simulink model "EPT"  (R2019b)
settings: Solver=FixedStepDiscrete  StartTime=0.0  StopTime=5  FixedStep=0.005  RelTol=1e-3  EnableMultiTasking=on
PreLoadFcn:
  | try, model_open; catch, disp('Error occurred while executing model pre-load callback: model_open.m'); disp('Please assure that the MATLAB working directory is set to the model directory before opening.'); end
InitFcn:
  | try, model_open; catch, end
undefined symbols (not defined in the file or in its folder): Bridge, GCM, H, ln, raptor_get_param_eval, raptor_get_safe_string, raptor_xcp_function
libraries: Raptor_lib x2810, simulink x374, hdlsllib x19
(part 9 of 45)

== system EPT/Foreground_TimeBase_5ms/CHG//DCHG_PW_Control/CHG//DCHG_Current_Control/Idchg_con Soft Recovery  ==
  Idch_con : Inport
  Constant : Constant
  Delay : Delay  DelayLength=1
  Delay1 : Subsystem
  Display{1..4} (4 alike) : Display
  Latch1 : Subsystem
  Logical Operator : Logic  Operator=OR  AllPortsSameDT=off  OutDataTypeStr=boolean
  NOT : Logic  Operator=NOT  IconShape=distinctive  AllPortsSameDT=off  OutDataTypeStr=boolean
  Product1 : Product
  Relational Operator1 : RelationalOperator  OutDataTypeStr=boolean  RndMeth=Simplest
  Saturation Dynamic2 : simulink/Discontinuities/Saturation Dynamic  OutMin=[]  OutMax=[]  OutDataTypeStr=Inherit: Same as second input  OutDataType=fixdt(1, 16)  OutScaling=2^-10  DoSatur=off
  Sum : Sum  Inputs=+-
  Sum1 : Sum
  Switch : Switch  Criteria=u2 > Threshold
      settings: LockScale=on
  Switch1 : Switch  Criteria=u2 > Threshold
      settings: LockScale=on
  raptor_adjustment1 : Raptor_lib/Data Storage/raptor_adjustment  paramName='Cal_Idschg_con_Soft_recovery_TimeCount'  nameSource=Parameter  initValue=3  dataType=double  storage=Calibration  calDispType=Number  calEnum={'False', 'True'}  calGain=1.0  calOffset=0.0  calMax=inf  calMin=-inf  calFormat='-1'  calUnit=''  calHelp=''  calAccess=1  calFunction=raptor_xcp_function(gcb)  calDispHeaders=off  calColHeaders={'Col1' 'Col2' 'Col3'}  calRowHeaders={'Row1' 'Row2' 'Row3'}
      settings: SourceProductName=Raptor
  raptor_adjustment2 : Raptor_lib/Data Storage/raptor_adjustment  paramName='Cal_Idschg_con_Soft_recovery_PID_offset'  nameSource=Parameter  initValue=-0.001  dataType=double  storage=Calibration  calDispType=Number  calEnum={'False', 'True'}  calGain=1.0  calOffset=0.0  calMax=inf  calMin=-inf  calFormat='-1'  calUnit=''  calHelp=''  calAccess=1  calFunction=raptor_xcp_function(gcb)  calDispHeaders=off  calColHeaders={'Col1' 'Col2' 'Col3'}  calRowHeaders={'Row1' 'Row2' 'Row3'}
      settings: SourceProductName=Raptor
  raptor_adjustment4 : Raptor_lib/Data Storage/raptor_adjustment  paramName='Cal_Idschg_con_Soft_recovery_PID_KI'  nameSource=Parameter  initValue=0.05  dataType=double  storage=Calibration  calDispType=Number  calEnum={'False', 'True'}  calGain=1.0  calOffset=0.0  calMax=inf  calMin=-inf  calFormat='-1'  calUnit=''  calHelp=''  calAccess=1  calFunction=raptor_xcp_function(gcb)  calDispHeaders=off  calColHeaders={'Col1' 'Col2' 'Col3'}  calRowHeaders={'Row1' 'Row2' 'Row3'}
      settings: SourceProductName=Raptor
  Idchg_con : Outport
  wires:
  Saturation Dynamic2/1 -> Display4/1, Sum1/1
  Idch_con/1 -> Switch/1, Product1/2, Sum/1, Switch1/1, Relational Operator1/1
  Sum/1 -> Display3/1
  Switch/1 -> Sum/2
  Product1/1 -> Saturation Dynamic2/2
  raptor_adjustment2/1 -> Saturation Dynamic2/3, Saturation Dynamic2/1
  Sum1/1 -> Delay/1
  raptor_adjustment4/1 -> Product1/1
  Switch1/1 -> Sum1/2, Display2/1, Display1/1, Idchg_con/1
  Delay/1 -> Switch1/3, Switch/3, Relational Operator1/2
  Relational Operator1/1 -> Logical Operator/1
  Constant/1 -> Delay1/1(Condition)
  Latch1/1(Output) -> NOT/1
  Logical Operator/1 -> Switch1/2, Switch/2
  raptor_adjustment1/1 -> Delay1/2(TimeCount)
  Delay1/1(Output) -> Latch1/1(Latch)
  NOT/1 -> Logical Operator/2

== system EPT/Foreground_TimeBase_5ms/CHG//DCHG_PW_Control/CHG//DCHG_Current_Control/Soft Recovery ==
  HV_Current : Inport
  Idchg_con : Inport  Port=2
  Add4 : Sum  Inputs=+-
  Delay : Delay  DelayLength=1
  Delay1 : Delay  DelayLength=1
  Gain1 : Gain  Gain=1.5
  IsNegative : simulink/Logic and Bit Operations/Compare To Zero  relop=<  OutDataTypeStr=boolean
  IsPositive : simulink/Logic and Bit Operations/Compare To Zero  relop=>  OutDataTypeStr=boolean
  Logical Operator3 : Logic  AllPortsSameDT=off  OutDataTypeStr=boolean
  Logical Operator4 : Logic  AllPortsSameDT=off  OutDataTypeStr=boolean
  Logical Operator5 : Logic  Operator=NOR  AllPortsSameDT=off  OutDataTypeStr=boolean
  Relational Operator2 : RelationalOperator  Operator=<=  OutDataTypeStr=boolean  RndMeth=Simplest
  Relational Operator3 : RelationalOperator  OutDataTypeStr=boolean  RndMeth=Simplest
  Saturation Dynamic2 : simulink/Discontinuities/Saturation Dynamic  OutMin=[]  OutMax=[]  OutDataTypeStr=Inherit: Same as second input  OutDataType=fixdt(1, 16)  OutScaling=2^-10  DoSatur=off
  Subsystem2 : Subsystem
  raptor_adjustment : Raptor_lib/Data Storage/raptor_adjustment  paramName='Cal_Recovery_Time_Ft'  nameSource=Parameter  initValue=0.066  dataType=double  storage=Calibration  calDispType=Number  calEnum={'False', 'True'}  calGain=1.0  calOffset=0.0  calMax=inf  calMin=-inf  calFormat='-1'  calUnit=''  calHelp=''  calAccess=1  calFunction=raptor_xcp_function(gcb)  calDispHeaders=off  calColHeaders={'Col1' 'Col2' 'Col3'}  calRowHeaders={'Row1' 'Row2' 'Row3'}
      settings: SourceProductName=Raptor
  Idchg_exp : Outport
  wires:
  Gain1/1 -> Saturation Dynamic2/3, Relational Operator2/2
  Idchg_con/1 -> Relational Operator3/2, Saturation Dynamic2/1, Gain1/1, Subsystem2/1(Idchg_con), Add4/2
  IsNegative/1 -> Logical Operator4/1
  Logical Operator4/1 -> Logical Operator5/2
  IsPositive/1 -> Logical Operator3/1
  Logical Operator5/1 -> Subsystem2/Enable
  Logical Operator3/1 -> Logical Operator5/1
  Relational Operator3/1 -> Delay1/1
  Saturation Dynamic2/1 -> Relational Operator2/1, Relational Operator3/1, Idchg_exp/1
  Subsystem2/1(Gain_Integral) -> Saturation Dynamic2/2
  Relational Operator2/1 -> Delay/1
  HV_Current/1 -> Add4/1
  raptor_adjustment/1 -> Subsystem2/3(Recovery_Time_Ft)
  Delay/1 -> Logical Operator3/2
  Delay1/1 -> Logical Operator4/2
  Add4/1 -> Subsystem2/2(Delta_Idchg), IsNegative/1, IsPositive/1

== system EPT/Foreground_TimeBase_5ms/CHG//DCHG_PW_Control/Coulomb Counting Algorithm/Coulomb Counting Algorithm ==
  Ampere input : Inport
  RC input : Inport  Port=2
  20ms : Subsystem
  Constant6 : Constant  Value=4
  CountTrigger : Subsystem
  wires:
  CountTrigger/1(Tirgger) -> 20ms/Trigger
  Constant6/1 -> CountTrigger/1(Counter)
  RC input/1 -> 20ms/2(RC input)
  Ampere input/1 -> 20ms/1(Ampere input)

== system EPT/Foreground_TimeBase_5ms/CHG//DCHG_PW_Control/Coulomb Counting Algorithm/Delay ==
  Condition : Inport
  TimeCount : Inport  Port=2
  Constant10 : Constant
  Constant11 : Constant  Value=0
  Constant8 : Constant  Value=0
  CycleTrigger : Subsystem
  Switch2 : Switch  Threshold=1
  Switch3 : Switch  Threshold=1
  Unit Delay1 : UnitDelay  SampleTime=-1  HasFrameUpgradeWarning=on
  Unit Delay2 : UnitDelay  SampleTime=-1  HasFrameUpgradeWarning=on
  Output : Outport  VectorParamsAs1DForOutWhenUnconnected=off
  wires:
  TimeCount/1 -> CycleTrigger/2(In2)
  Condition/1 -> Switch3/2
  CycleTrigger/1(Trigger) -> Switch2/2, Unit Delay1/1
  Constant8/1 -> Switch2/1
  Constant10/1 -> Switch2/3
  Switch3/1 -> CycleTrigger/1(In1)
  Constant11/1 -> Switch3/3
  Unit Delay2/1 -> Switch3/1
  Switch2/1 -> Unit Delay2/1
  Unit Delay1/1 -> Output/1

== system EPT/Foreground_TimeBase_5ms/CHG//DCHG_PW_Control/Coulomb Counting Algorithm/Latch ==
  Latch : Inport
  Reset : Inport  Port=2
  Switch1 : Switch  Criteria=u2 > Threshold
  Switch3 : Switch  Criteria=u2 > Threshold
  Unit Delay1 : UnitDelay  SampleTime=-1  HasFrameUpgradeWarning=on
  Output : Outport  VectorParamsAs1DForOutWhenUnconnected=off
  wires:
  Unit Delay1/1 -> Switch1/3
  Switch3/1 -> Output/1, Unit Delay1/1
  Reset/1 -> Switch3/2
  Latch/1 -> Switch1/1, Switch1/2
  Switch1/1 -> Switch3/3

== system EPT/Foreground_TimeBase_5ms/CHG//DCHG_PW_Control/Coulomb Counting Algorithm/WH  ==
  Ampere input : Inport
  Voltage input : Inport  Port=2
  WH input : Inport  Port=3
  Enable : EnablePort
  20ms : Subsystem
  Constant6 : Constant  Value=4
  CountTrigger : Subsystem
  WH Output : Outport  VectorParamsAs1DForOutWhenUnconnected=off
  wires:
  Voltage input/1 -> 20ms/2(Voltage input)
  Ampere input/1 -> 20ms/1(Ampere input)
  20ms/1(WH Output) -> WH Output/1
  Constant6/1 -> CountTrigger/1(Counter)
  CountTrigger/1(Tirgger) -> 20ms/Trigger
  WH input/1 -> 20ms/3(WH Input)

== system EPT/Foreground_TimeBase_5ms/CHG//DCHG_PW_Control/EOC/Delay1 ==
  Condition : Inport
  TimeCount : Inport  Port=2
  Constant10 : Constant
  Constant11 : Constant  Value=0
  Constant8 : Constant  Value=0
  CycleTrigger : Subsystem
  Switch2 : Switch  Threshold=1
  Switch3 : Switch  Threshold=1
  Unit Delay1 : UnitDelay  SampleTime=-1  HasFrameUpgradeWarning=on
  Unit Delay2 : UnitDelay  SampleTime=-1  HasFrameUpgradeWarning=on
  Output : Outport  VectorParamsAs1DForOutWhenUnconnected=off
  wires:
  Unit Delay1/1 -> Output/1
  Switch2/1 -> Unit Delay2/1
  Unit Delay2/1 -> Switch3/1
  Constant11/1 -> Switch3/3
  Switch3/1 -> CycleTrigger/1(In1)
  Constant10/1 -> Switch2/3
  Constant8/1 -> Switch2/1
  CycleTrigger/1(Trigger) -> Unit Delay1/1, Switch2/2
  Condition/1 -> Switch3/2
  TimeCount/1 -> CycleTrigger/2(In2)

== system EPT/Foreground_TimeBase_5ms/CHG//DCHG_PW_Control/EOC/EOC_Table ==
  Abs : Abs
  Add : Sum
  raptor_adjustment1 : Raptor_lib/Data Storage/raptor_adjustment  paramName='EOC_Offset'  nameSource=Parameter  initValue=0.0  dataType=double  storage=Calibration  calDispType=Number  calEnum={'False', 'True'}  calGain=1.0  calOffset=0.0  calMax=inf  calMin=-inf  calFormat='-1'  calUnit=''  calHelp=''  calAccess=1  calFunction=raptor_xcp_function(gcb)  calDispHeaders=off  calColHeaders={'Col1' 'Col2' 'Col3'}  calRowHeaders={'Row1' 'Row2' 'Row3'}
      settings: SourceProductName=Raptor
  raptor_data_read9 : Raptor_lib/Data Storage/raptor_data_read  dataName='EPT_BPOBU_CURR'  dataShape=Scalar  idxSource=Input  idxRow=1  idxCol=1
      settings: SourceProductName=Raptor
  raptor_table_1d1 : Raptor_lib/Table Lookup/raptor_table_1d  dataName='Amp2EOCVoltage_V2'  initValue=|  dataType=double  storage=Calibration  initValueX=|  dataTypeXY=double  storageXY=Calibration  calVisible=on  showTable=on  calGain=1  calOffset=0.0  calMax=Inf  calMin=-Inf  calFormat='-1'  calUnit=''  calHelp=''  showBreakpoint=on  dataNameX=[]  calGainX=1.0  calOffsetX=0.0  calMaxX=Inf  calMinX=-Inf  calFormatX='-1'  calUnitX=''  calHelpX=''  calAccess=1  calFunction=raptor_xcp_function(gcb)  measureEnable=off  mName=[raptor_get_param_eval(gcb,'dataName'), '_Output']
      initValue=|
      | [3.4
      | 3.45
      | 3.48
      | 3.5
      | 3.52
      | 3.54
      | 3.56
      | 3.58
      | 3.6
      | ]
      initValueX=|
      | [0
      | 5
      | 10
      | 15
      | 20
      | 25
      | 30
      | 40
      | 50
      | ]
      settings: SourceProductName=Raptor
  raptor_table_1d2 : Raptor_lib/Table Lookup/raptor_table_1d  dataName='Amp2EOCVoltage'  initValue=|  dataType=double  storage=Calibration  initValueX=|  dataTypeXY=double  storageXY=Calibration  calVisible=on  showTable=on  calGain=1  calOffset=0.0  calMax=Inf  calMin=-Inf  calFormat='-1'  calUnit=''  calHelp=''  showBreakpoint=on  dataNameX=[]  calGainX=1.0  calOffsetX=0.0  calMaxX=Inf  calMinX=-Inf  calFormatX='-1'  calUnitX=''  calHelpX=''  calAccess=1  calFunction=raptor_xcp_function(gcb)  measureEnable=off  mName=[raptor_get_param_eval(gcb,'dataName'), '_Output']
      initValue=|
      | [3.34
      | 3.35
      | 3.36
      | 3.39
      | 3.4
      | 3.41
      | 3.42
      | 3.45
      | 3.5
      | 3.5
      | 3.5
      | 3.5
      | 
      | ]
      initValueX=|
      | [0
      | 2.5
      | 5
      | 7.5
      | 10
      | 12.5
      | 15
      | 20
      | 25
      | 37.5
      | 50
      | 100
      | ]*3
      settings: SourceProductName=Raptor
  CellVoltage : Outport  VectorParamsAs1DForOutWhenUnconnected=off
  wires:
  raptor_table_1d1/1 -> Add/1
  raptor_adjustment1/1 -> Add/2
  raptor_data_read9/1 -> Abs/1
  Add/1 -> CellVoltage/1
  Abs/1 -> raptor_table_1d1/1

== system EPT/Foreground_TimeBase_5ms/CHG//DCHG_PW_Control/EOC/Latch1 ==
  Latch : Inport
  Reset : Inport  Port=2
  Switch1 : Switch  Criteria=u2 > Threshold
  Switch3 : Switch  Criteria=u2 > Threshold
  Unit Delay1 : UnitDelay  SampleTime=-1  HasFrameUpgradeWarning=on
  Output : Outport  VectorParamsAs1DForOutWhenUnconnected=off
  wires:
  Unit Delay1/1 -> Switch1/3
  Switch3/1 -> Output/1, Unit Delay1/1
  Reset/1 -> Switch3/2
  Latch/1 -> Switch1/1, Switch1/2
  Switch1/1 -> Switch3/3

== system EPT/Foreground_TimeBase_5ms/CHG//DCHG_PW_Control/EOD/Delay1 ==
  Condition : Inport
  TimeCount : Inport  Port=2
  Constant10 : Constant
  Constant11 : Constant  Value=0
  Constant8 : Constant  Value=0
  CycleTrigger : Subsystem
  Switch2 : Switch  Threshold=1
  Switch3 : Switch  Threshold=1
  Unit Delay1 : UnitDelay  SampleTime=-1  HasFrameUpgradeWarning=on
  Unit Delay2 : UnitDelay  SampleTime=-1  HasFrameUpgradeWarning=on
  Output : Outport  VectorParamsAs1DForOutWhenUnconnected=off
  wires:
  Unit Delay1/1 -> Output/1
  Switch2/1 -> Unit Delay2/1
  Unit Delay2/1 -> Switch3/1
  Constant11/1 -> Switch3/3
  Switch3/1 -> CycleTrigger/1(In1)
  Constant10/1 -> Switch2/3
  Constant8/1 -> Switch2/1
  CycleTrigger/1(Trigger) -> Unit Delay1/1, Switch2/2
  Condition/1 -> Switch3/2
  TimeCount/1 -> CycleTrigger/2(In2)

== system EPT/Foreground_TimeBase_5ms/CHG//DCHG_PW_Control/EOD/EOD_Table ==
  Abs : Abs
  Display : Display
  Subtract : Sum  Inputs=+-
  raptor_adjustment : Raptor_lib/Data Storage/raptor_adjustment  paramName='EOD_Offset'  nameSource=Parameter  initValue=0.1  dataType=double  storage=Calibration  calDispType=Number  calEnum={'False', 'True'}  calGain=1.0  calOffset=0.0  calMax=inf  calMin=-inf  calFormat='-1'  calUnit=''  calHelp=''  calAccess=1  calFunction=raptor_xcp_function(gcb)  calDispHeaders=off  calColHeaders={'Col1' 'Col2' 'Col3'}  calRowHeaders={'Row1' 'Row2' 'Row3'}
      settings: SourceProductName=Raptor
  raptor_data_read9 : Raptor_lib/Data Storage/raptor_data_read  dataName='EPT_BPOBU_CURR'  dataShape=Scalar  idxSource=Input  idxRow=1  idxCol=1
      settings: SourceProductName=Raptor
  raptor_table_1d1 : Raptor_lib/Table Lookup/raptor_table_1d  dataName='Amp2EODVoltage'  initValue=|  dataType=double  storage=Calibration  initValueX=|  dataTypeXY=double  storageXY=Calibration  calVisible=on  showTable=on  calGain=1  calOffset=0.0  calMax=Inf  calMin=-Inf  calFormat='-1'  calUnit=''  calHelp=''  showBreakpoint=on  dataNameX=[]  calGainX=1.0  calOffsetX=0.0  calMaxX=Inf  calMinX=-Inf  calFormatX='-1'  calUnitX=''  calHelpX=''  calAccess=1  calFunction=raptor_xcp_function(gcb)  measureEnable=off  mName=[raptor_get_param_eval(gcb,'dataName'), '_Output']
      initValue=|
      | [3.05
      | 2.99
      | 2.94
      | 2.89
      | 2.86
      | 2.82
      | 2.79
      | 2.72
      | 2.65
      | 2.6
      | 2.6
      | 2.6
      | 2.6
      | ]
      initValueX=|
      | [0
      | 5
      | 10
      | 15
      | 20
      | 25
      | 30
      | 40
      | 50
      | 100
      | 150
      | 200
      | 300
      | ]
      settings: SourceProductName=Raptor
  CellVoltage : Outport  VectorParamsAs1DForOutWhenUnconnected=off
  wires:
  Subtract/1 -> CellVoltage/1, Display/1
  raptor_table_1d1/1 -> Subtract/1
  raptor_adjustment/1 -> Subtract/2
  raptor_data_read9/1 -> Abs/1
  Abs/1 -> raptor_table_1d1/1

== system EPT/Foreground_TimeBase_5ms/CHG//DCHG_PW_Control/EOD/Latch1 ==
  Latch : Inport
  Reset : Inport  Port=2
  Switch1 : Switch  Criteria=u2 > Threshold
  Switch3 : Switch  Criteria=u2 > Threshold
  Unit Delay1 : UnitDelay  SampleTime=-1  HasFrameUpgradeWarning=on
  Output : Outport  VectorParamsAs1DForOutWhenUnconnected=off
  wires:
  Unit Delay1/1 -> Switch1/3
  Switch3/1 -> Output/1, Unit Delay1/1
  Reset/1 -> Switch3/2
  Latch/1 -> Switch1/1, Switch1/2
  Switch1/1 -> Switch3/3

== system EPT/Foreground_TimeBase_5ms/CHG//DCHG_PW_Control/Enhanced Coulomb Counting Algorithm/Coulomb Counting ==
  Ib : Inport
  Ah Input : Inport  Port=2
  20ms : Subsystem
  Constant6 : Constant  Value=4
  CountTrigger : Subsystem
  Gain2 : Gain  Gain=-1
  Ah Output : Outport
  wires:
  Ah Input/1 -> 20ms/2(Delta_DoD)
  Constant6/1 -> CountTrigger/1(Counter)
  CountTrigger/1(Tirgger) -> 20ms/Trigger
  20ms/1(Delta DoD) -> Ah Output/1
  Ib/1 -> Gain2/1
  Gain2/1 -> 20ms/1(Ib)

== system EPT/Foreground_TimeBase_5ms/CHG//DCHG_PW_Control/Enhanced Coulomb Counting Algorithm/Init Enhanced Coulomb Counting Algorithm ==
  Enable : EnablePort
  raptor_adjustment : Raptor_lib/Data Storage/raptor_adjustment  paramName='Cal_DOD_t0'  nameSource=Parameter  initValue=0.00  dataType=double  storage=Calibration  calDispType=Number  calEnum={'False', 'True'}  calGain=1.0  calOffset=0.0  calMax=inf  calMin=-inf  calFormat='-1'  calUnit=''  calHelp=''  calAccess=1  calFunction=raptor_xcp_function(gcb)  calDispHeaders=off  calColHeaders={'Col1' 'Col2' 'Col3'}  calRowHeaders={'Row1' 'Row2' 'Row3'}
      settings: SourceProductName=Raptor
  raptor_adjustment1 : Raptor_lib/Data Storage/raptor_adjustment  paramName='Cal_SOH'  nameSource=Parameter  initValue=0.00  dataType=double  storage=Calibration  calDispType=Number  calEnum={'False', 'True'}  calGain=1.0  calOffset=0.0  calMax=inf  calMin=-inf  calFormat='-1'  calUnit=''  calHelp=''  calAccess=1  calFunction=raptor_xcp_function(gcb)  calDispHeaders=off  calColHeaders={'Col1' 'Col2' 'Col3'}  calRowHeaders={'Row1' 'Row2' 'Row3'}
      settings: SourceProductName=Raptor
  raptor_data_write1 : Raptor_lib/Data Storage/raptor_data_write  dataName='SOH'  dataShape=Scalar  idxSource=Input Port  idxRow=1  idxCol=1
      settings: SourceProductName=Raptor
  raptor_data_write2 : Raptor_lib/Data Storage/raptor_data_write  dataName='DOD_t0'  dataShape=Scalar  idxSource=Input Port  idxRow=1  idxCol=1
      settings: SourceProductName=Raptor
  wires:
  raptor_adjustment/1 -> raptor_data_write2/1
  raptor_adjustment1/1 -> raptor_data_write1/1

== system EPT/Foreground_TimeBase_5ms/CHG//DCHG_PW_Control/Enhanced Coulomb Counting Algorithm Backup/Coulomb Counting1 ==
  Ib : Inport
  Ah Input : Inport  Port=2
  20ms : Subsystem
  Constant6 : Constant  Value=4
  CountTrigger : Subsystem
  Gain2 : Gain  Gain=-1
  Ah Output : Outport
  wires:
  Gain2/1 -> 20ms/1(Ib)
  Ib/1 -> Gain2/1
  20ms/1(Delta DoD) -> Ah Output/1
  CountTrigger/1(Tirgger) -> 20ms/Trigger
  Constant6/1 -> CountTrigger/1(Counter)
  Ah Input/1 -> 20ms/2(Delta_DoD)

== system EPT/Foreground_TimeBase_5ms/CHG//DCHG_PW_Control/SWU Power Divider/PWCU ==
  Constant1 : Constant
  Constant10 : Constant  Value=70
  Constant3 : Constant  Value=50
  Constant9 : Constant
  Latch1 : Subsystem
  Latch2 : Subsystem
  Product{2..6} (5 alike) : Product
  Relational Operator1 : RelationalOperator  Operator=>  OutDataTypeStr=boolean  RndMeth=Simplest
  Relational Operator2 : RelationalOperator  Operator=>  OutDataTypeStr=boolean  RndMeth=Simplest
  Relational Operator3 : RelationalOperator  Operator=<=  OutDataTypeStr=boolean  RndMeth=Simplest
  Relational Operator4 : RelationalOperator  Operator=<=  OutDataTypeStr=boolean  RndMeth=Simplest
  Saturation Dynamic : simulink/Discontinuities/Saturation Dynamic  OutMin=[]  OutMax=[]  OutDataTypeStr=Inherit: Same as second input  OutDataType=fixdt(1, 16)  OutScaling=2^-10  DoSatur=off
  Subtract3 : Sum
  Subtract4 : Sum  Inputs=+-
  Subtract5 : Sum
  Subtract6 : Sum  Inputs=+-
  Switch1 : Switch  Criteria=u2 > Threshold
  Total PW. : Constant  Value=9
  raptor_adjustment : Raptor_lib/Data Storage/raptor_adjustment  paramName='Cal_OBU_RSOC_Lower_Limit_error'  nameSource=Parameter  initValue=0.02  dataType=double  storage=Calibration  calDispType=Number  calEnum={'False', 'True'}  calGain=1.0  calOffset=0.0  calMax=inf  calMin=-inf  calFormat='-1'  calUnit=''  calHelp=''  calAccess=1  calFunction=raptor_xcp_function(gcb)  calDispHeaders=off  calColHeaders={'Col1' 'Col2' 'Col3'}  calRowHeaders={'Row1' 'Row2' 'Row3'}
      settings: SourceProductName=Raptor
  raptor_adjustment2 : Raptor_lib/Data Storage/raptor_adjustment  paramName='Cal_OBU_RSOC_Upper_Limit_error'  nameSource=Parameter  initValue=0.02  dataType=double  storage=Calibration  calDispType=Number  calEnum={'False', 'True'}  calGain=1.0  calOffset=0.0  calMax=inf  calMin=-inf  calFormat='-1'  calUnit=''  calHelp=''  calAccess=1  calFunction=raptor_xcp_function(gcb)  calDispHeaders=off  calColHeaders={'Col1' 'Col2' 'Col3'}  calRowHeaders={'Row1' 'Row2' 'Row3'}
      settings: SourceProductName=Raptor
  raptor_data_read1 : Raptor_lib/Data Storage/raptor_data_read  dataName='SWCU_BPSWU_POUT_MAX'  dataShape=Scalar  idxSource=Input  idxRow=1  idxCol=1
      settings: SourceProductName=Raptor
  raptor_data_read3 : Raptor_lib/Data Storage/raptor_data_read  dataName='EPT_BPOBU_SOC'  dataShape=Scalar  idxSource=Input  idxRow=1  idxCol=1
      settings: SourceProductName=Raptor
  raptor_data_write7 : Raptor_lib/Data Storage/raptor_data_write  dataName='EPT_SWCU_POUT_CMD'  dataShape=Scalar  idxSource=Input Port  idxRow=1  idxCol=1
      settings: SourceProductName=Raptor
  raptor_override3 : Raptor_lib/Data Storage/raptor_override  paramName='Cal_OBU_ROSC'  nameSource=Parameter  measurement=None  calDispType=Number  calEnum={'False', 'True'}  calGain=1.0  calOffset=0.0  calMax=inf  calMin=-inf  calFormat='-1'  calUnit=''  calHelp=''  calAccess=1  calFunction=[raptor_xcp_function(gcb) '|' raptor_get_param_eval(gcb, 'paramName') '_Override']
      settings: SourceProductName=Raptor
  raptor_table_1d : Raptor_lib/Table Lookup/raptor_table_1d  dataName='OBU_SOC2SWCU_PW'  initValue="[9 9 7.5  7.5 3.6 3.6 3.6]"  dataType=double  storage=Calibration  initValueX=[0 50 50 55 65 70 75]  dataTypeXY=double  storageXY=Calibration  calVisible=on  showTable=on  calGain=1.0  calOffset=0.0  calMax=Inf  calMin=-Inf  calFormat='-1'  calUnit=''  calHelp=''  showBreakpoint=on  dataNameX=[]  calGainX=1.0  calOffsetX=0.0  calMaxX=Inf  calMinX=-Inf  calFormatX='-1'  calUnitX=''  calHelpX=''  calAccess=1  calFunction=raptor_xcp_function(gcb)  measureEnable=off  mName=[raptor_get_param_eval(gcb,'dataName'), '_Output']
      settings: SourceProductName=Raptor
  wires:
  Product5/1 -> Relational Operator4/2
  Relational Operator3/1 -> Latch1/1(Latch)
  Product4/1 -> Relational Operator1/2
  Subtract3/1 -> Product4/2
  Relational Operator4/1 -> Latch2/1(Latch)
  Product3/1 -> Relational Operator3/2
  raptor_adjustment/1 -> Subtract3/2, Subtract4/2
  raptor_adjustment2/1 -> Subtract5/2, Subtract6/2
  Relational Operator1/1 -> Latch1/2(Reset)
  Latch2/1(Output) -> Product2/2
  Product2/1 -> Switch1/3
  Constant9/1 -> Subtract5/1, Subtract6/1
  raptor_override3/1 -> Relational Operator2/1, Relational Operator4/1, Relational Operator3/1, Relational Operator1/1, raptor_table_1d/1
  Relational Operator2/1 -> Latch2/2(Reset)
  raptor_data_read3/1 -> raptor_override3/1
  Constant3/1 -> Product4/1, Product3/1
  Subtract6/1 -> Product5/2
  raptor_table_1d/1 -> Product2/1
  Constant10/1 -> Product6/1, Product5/1
  Product6/1 -> Relational Operator2/2
  Subtract5/1 -> Product6/2
  Subtract4/1 -> Product3/2
  Latch1/1(Output) -> Switch1/2
  Total PW./1 -> Switch1/1
  Constant1/1 -> Subtract3/1, Subtract4/1
  Switch1/1 -> Saturation Dynamic/2
  Saturation Dynamic/1 -> raptor_data_write7/1
  raptor_data_read1/1 -> Saturation Dynamic/1

== system EPT/Foreground_TimeBase_5ms/E//W /BP-OBU_E//W/BP-OBU_E//W ==
  "CMU_Work " : Inport
  BP-OBU_Fault_G4 : Subsystem
  BP-OBU_Warning/Fault_G1 : Subsystem
  BP-OBU_Warning/Fault_G2 : Subsystem
  BP-OBU_Warning/Fault_G3 : Subsystem
  BP-OBU_Warning/Fault_G5 : Subsystem
  wires:
  "CMU_Work "/1 -> BP-OBU_Fault_G4/1("CMU_Work "), BP-OBU_Warning/Fault_G2/Enable, BP-OBU_Warning/Fault_G1/Enable

== system EPT/Foreground_TimeBase_5ms/E//W /BP-OBU_E//W/Delay ==
  Condition : Inport
  TimeCount : Inport  Port=2
  Constant10 : Constant
  Constant11 : Constant  Value=0
  Constant8 : Constant  Value=0
  CycleTrigger : Subsystem
  Switch2 : Switch  Threshold=1
  Switch3 : Switch  Threshold=1
  Unit Delay1 : UnitDelay  SampleTime=-1  HasFrameUpgradeWarning=on
  Unit Delay2 : UnitDelay  SampleTime=-1  HasFrameUpgradeWarning=on
  Output : Outport  VectorParamsAs1DForOutWhenUnconnected=off
  wires:
  TimeCount/1 -> CycleTrigger/2(In2)
  Condition/1 -> Switch3/2
  CycleTrigger/1(Trigger) -> Switch2/2, Unit Delay1/1
  Constant8/1 -> Switch2/1
  Constant10/1 -> Switch2/3
  Switch3/1 -> CycleTrigger/1(In1)
  Constant11/1 -> Switch3/3
  Unit Delay2/1 -> Switch3/1
  Switch2/1 -> Unit Delay2/1
  Unit Delay1/1 -> Output/1

== system EPT/Foreground_TimeBase_5ms/E//W /BP-OBU_E//W/Latch ==
  Latch : Inport
  Reset : Inport  Port=2
  Switch1 : Switch  Criteria=u2 > Threshold
  Switch3 : Switch  Criteria=u2 > Threshold
  Unit Delay1 : UnitDelay  SampleTime=-1  HasFrameUpgradeWarning=on
  Output : Outport  VectorParamsAs1DForOutWhenUnconnected=off
  wires:
  Unit Delay1/1 -> Switch1/3
  Switch3/1 -> Output/1, Unit Delay1/1
  Reset/1 -> Switch3/2
  Latch/1 -> Switch1/1, Switch1/2
  Switch1/1 -> Switch3/3

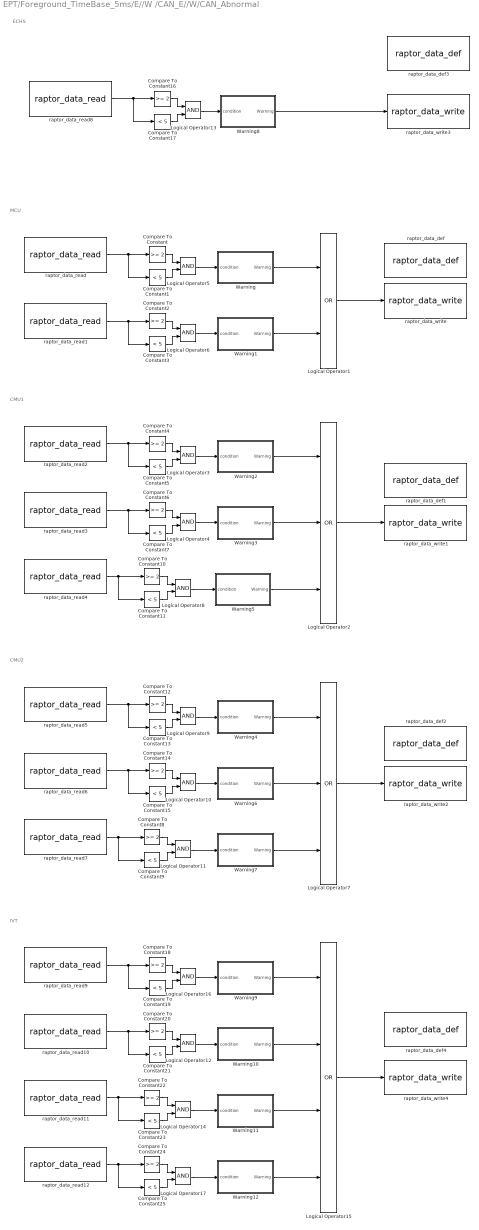
== system EPT/Foreground_TimeBase_5ms/E//W /CAN_E//W/CAN_Abnormal ==
  note: MCU
  note: CMU1
  note: CMU2
  note: ECHS
  note: IVT
  Compare To Constant{,2,4,6,8,10,12,14,16,18,20,22,24} (13 alike) : simulink/Logic and Bit Operations/Compare To Constant  relop=>=  const=2  OutDataTypeStr=boolean
  Compare To Constant{1,3,5,7,9,11,13,15,17,19,21,23,25} (13 alike) : simulink/Logic and Bit Operations/Compare To Constant  relop=<  const=5  OutDataTypeStr=boolean
  Logical Operator1 : Logic  Operator=OR  AllPortsSameDT=off  OutDataTypeStr=boolean
  Logical Operator{3..6,8..14,16..17} (13 alike) : Logic  AllPortsSameDT=off  OutDataTypeStr=boolean
  Logical Operator15 : Logic  Operator=OR  Inputs=4  AllPortsSameDT=off  OutDataTypeStr=boolean
  Logical Operator2 : Logic  Operator=OR  Inputs=3  AllPortsSameDT=off  OutDataTypeStr=boolean
  Logical Operator7 : Logic  Operator=OR  Inputs=3  AllPortsSameDT=off  OutDataTypeStr=boolean
  Warning : Subsystem
  Warning1 : Subsystem
  Warning10 : Subsystem
  Warning11 : Subsystem
  Warning12 : Subsystem
  Warning2 : Subsystem
  Warning3 : Subsystem
  Warning4 : Subsystem
  Warning5 : Subsystem
  Warning6 : Subsystem
  Warning7 : Subsystem
  Warning8 : Subsystem
  Warning9 : Subsystem
  raptor_data_def : Raptor_lib/Data Storage/raptor_data_def  dataName='CAN_Abnormal_MCU'  initValue=0  dataType=boolean  storage=Volatile (RAM)  calVisible=on  calType=Measurement  calDispType=Number  calEnum={'False', 'True'}  calGain=1.0  calOffset=0  calMin=-inf  calMax=inf  calFormat='-1'  calUnit=''  calHelp=''  calAccess=1  calFunction=raptor_xcp_function(gcb)  calDispHeaders=off  calColHeaders={'Col1' 'Col2' 'Col3'}  calRowHeaders={'Row1' 'Row2' 'Row3'}
      settings: SourceProductName=Raptor
  raptor_data_def1 : Raptor_lib/Data Storage/raptor_data_def  dataName='CAN_Abnormal_CMU1'  initValue=0  dataType=boolean  storage=Volatile (RAM)  calVisible=on  calType=Measurement  calDispType=Number  calEnum={'False', 'True'}  calGain=1.0  calOffset=0  calMin=-inf  calMax=inf  calFormat='-1'  calUnit=''  calHelp=''  calAccess=1  calFunction=raptor_xcp_function(gcb)  calDispHeaders=off  calColHeaders={'Col1' 'Col2' 'Col3'}  calRowHeaders={'Row1' 'Row2' 'Row3'}
      settings: SourceProductName=Raptor
  raptor_data_def2 : Raptor_lib/Data Storage/raptor_data_def  dataName='CAN_Abnormal_CMU2'  initValue=0  dataType=boolean  storage=Volatile (RAM)  calVisible=on  calType=Measurement  calDispType=Number  calEnum={'False', 'True'}  calGain=1.0  calOffset=0  calMin=-inf  calMax=inf  calFormat='-1'  calUnit=''  calHelp=''  calAccess=1  calFunction=raptor_xcp_function(gcb)  calDispHeaders=off  calColHeaders={'Col1' 'Col2' 'Col3'}  calRowHeaders={'Row1' 'Row2' 'Row3'}
      settings: SourceProductName=Raptor
  raptor_data_def3 : Raptor_lib/Data Storage/raptor_data_def  dataName='CAN_Abnormal_ECHS'  initValue=0  dataType=boolean  storage=Volatile (RAM)  calVisible=on  calType=Measurement  calDispType=Number  calEnum={'False', 'True'}  calGain=1.0  calOffset=0  calMin=-inf  calMax=inf  calFormat='-1'  calUnit=''  calHelp=''  calAccess=1  calFunction=raptor_xcp_function(gcb)  calDispHeaders=off  calColHeaders={'Col1' 'Col2' 'Col3'}  calRowHeaders={'Row1' 'Row2' 'Row3'}
      settings: SourceProductName=Raptor
  raptor_data_def4 : Raptor_lib/Data Storage/raptor_data_def  dataName='CAN_Abnormal_IVT'  initValue=0  dataType=boolean  storage=Volatile (RAM)  calVisible=on  calType=Measurement  calDispType=Number  calEnum={'False', 'True'}  calGain=1.0  calOffset=0  calMin=-inf  calMax=inf  calFormat='-1'  calUnit=''  calHelp=''  calAccess=1  calFunction=raptor_xcp_function(gcb)  calDispHeaders=off  calColHeaders={'Col1' 'Col2' 'Col3'}  calRowHeaders={'Row1' 'Row2' 'Row3'}
      settings: SourceProductName=Raptor
  raptor_data_read : Raptor_lib/Data Storage/raptor_data_read  dataName='Rx0x220_Age'  dataShape=Scalar  idxSource=Input  idxRow=1  idxCol=1
      settings: SourceProductName=Raptor
  raptor_data_read1 : Raptor_lib/Data Storage/raptor_data_read  dataName='Rx0x221_Age'  dataShape=Scalar  idxSource=Input  idxRow=1  idxCol=1
      settings: SourceProductName=Raptor
  raptor_data_read10 : Raptor_lib/Data Storage/raptor_data_read  dataName='Age_0x522'  dataShape=Scalar  idxSource=Input  idxRow=1  idxCol=1
      settings: SourceProductName=Raptor
  raptor_data_read11 : Raptor_lib/Data Storage/raptor_data_read  dataName='Age_0x523'  dataShape=Scalar  idxSource=Input  idxRow=1  idxCol=1
      settings: SourceProductName=Raptor
  raptor_data_read12 : Raptor_lib/Data Storage/raptor_data_read  dataName='Age_0x524'  dataShape=Scalar  idxSource=Input  idxRow=1  idxCol=1
      settings: SourceProductName=Raptor
  raptor_data_read2 : Raptor_lib/Data Storage/raptor_data_read  dataName='Rx0x200B0A1_Age'  dataShape=Scalar  idxSource=Input  idxRow=1  idxCol=1
      settings: SourceProductName=Raptor
  raptor_data_read3 : Raptor_lib/Data Storage/raptor_data_read  dataName='Rx0x200B1A1_Age'  dataShape=Scalar  idxSource=Input  idxRow=1  idxCol=1
      settings: SourceProductName=Raptor
  raptor_data_read4 : Raptor_lib/Data Storage/raptor_data_read  dataName='Rx0x200BAA1_Age'  dataShape=Scalar  idxSource=Input  idxRow=1  idxCol=1
      settings: SourceProductName=Raptor
  raptor_data_read5 : Raptor_lib/Data Storage/raptor_data_read  dataName='Rx0x200B0A2_Age'  dataShape=Scalar  idxSource=Input  idxRow=1  idxCol=1
      settings: SourceProductName=Raptor
  raptor_data_read6 : Raptor_lib/Data Storage/raptor_data_read  dataName='Rx0x200B2A2_Age'  dataShape=Scalar  idxSource=Input  idxRow=1  idxCol=1
      settings: SourceProductName=Raptor
  raptor_data_read7 : Raptor_lib/Data Storage/raptor_data_read  dataName='Rx0x200BBA2_Age'  dataShape=Scalar  idxSource=Input  idxRow=1  idxCol=1
      settings: SourceProductName=Raptor
  raptor_data_read8 : Raptor_lib/Data Storage/raptor_data_read  dataName='Rx0xC10F4D0_Age'  dataShape=Scalar  idxSource=Input  idxRow=1  idxCol=1
      settings: SourceProductName=Raptor
  raptor_data_read9 : Raptor_lib/Data Storage/raptor_data_read  dataName='Age_0x521'  dataShape=Scalar  idxSource=Input  idxRow=1  idxCol=1
      settings: SourceProductName=Raptor
  raptor_data_write : Raptor_lib/Data Storage/raptor_data_write  dataName='CAN_Abnormal_MCU'  dataShape=Scalar  idxSource=Input Port  idxRow=1  idxCol=1
      settings: SourceProductName=Raptor
  raptor_data_write1 : Raptor_lib/Data Storage/raptor_data_write  dataName='CAN_Abnormal_CMU1'  dataShape=Scalar  idxSource=Input Port  idxRow=1  idxCol=1
      settings: SourceProductName=Raptor
  raptor_data_write2 : Raptor_lib/Data Storage/raptor_data_write  dataName='CAN_Abnormal_CMU2'  dataShape=Scalar  idxSource=Input Port  idxRow=1  idxCol=1
      settings: SourceProductName=Raptor
  raptor_data_write3 : Raptor_lib/Data Storage/raptor_data_write  dataName='CAN_Abnormal_ECHS'  dataShape=Scalar  idxSource=Input Port  idxRow=1  idxCol=1
      settings: SourceProductName=Raptor
  raptor_data_write4 : Raptor_lib/Data Storage/raptor_data_write  dataName='CAN_Abnormal_IVT'  dataShape=Scalar  idxSource=Input Port  idxRow=1  idxCol=1
      settings: SourceProductName=Raptor
  wires:
  Compare To Constant/1 -> Logical Operator5/1
  Compare To Constant1/1 -> Logical Operator5/2
  raptor_data_read/1 -> Compare To Constant1/1, Compare To Constant/1
  raptor_data_read1/1 -> Compare To Constant3/1, Compare To Constant2/1
  Compare To Constant3/1 -> Logical Operator6/2
  Compare To Constant2/1 -> Logical Operator6/1
  Logical Operator5/1 -> Warning/1(" condition")
  Logical Operator6/1 -> Warning1/1(" condition")
  Warning/1(Warning) -> Logical Operator1/1
  Warning1/1(Warning) -> Logical Operator1/2
  Logical Operator1/1 -> raptor_data_write/1
  Logical Operator2/1 -> raptor_data_write1/1
  Warning3/1(Warning) -> Logical Operator2/2
  Warning2/1(Warning) -> Logical Operator2/1
  Logical Operator4/1 -> Warning3/1(" condition")
  Logical Operator3/1 -> Warning2/1(" condition")
  Compare To Constant6/1 -> Logical Operator4/1
  Compare To Constant7/1 -> Logical Operator4/2
  raptor_data_read3/1 -> Compare To Constant6/1, Compare To Constant7/1
  raptor_data_read2/1 -> Compare To Constant4/1, Compare To Constant5/1
  Compare To Constant5/1 -> Logical Operator3/2
  Compare To Constant4/1 -> Logical Operator3/1
  Warning5/1(Warning) -> Logical Operator2/3
  Logical Operator8/1 -> Warning5/1(" condition")
  Compare To Constant10/1 -> Logical Operator8/1
  Compare To Constant11/1 -> Logical Operator8/2
  raptor_data_read4/1 -> Compare To Constant10/1, Compare To Constant11/1
  Warning7/1(Warning) -> Logical Operator7/3
  raptor_data_read7/1 -> Compare To Constant8/1, Compare To Constant9/1
  raptor_data_read5/1 -> Compare To Constant12/1, Compare To Constant13/1
  Compare To Constant13/1 -> Logical Operator9/2
  Compare To Constant12/1 -> Logical Operator9/1
  Logical Operator10/1 -> Warning6/1(" condition")
  Warning4/1(Warning) -> Logical Operator7/1
  Compare To Constant15/1 -> Logical Operator10/2
  Warning6/1(Warning) -> Logical Operator7/2
  Logical Operator7/1 -> raptor_data_write2/1
  Logical Operator11/1 -> Warning7/1(" condition")
  Compare To Constant14/1 -> Logical Operator10/1
  Logical Operator9/1 -> Warning4/1(" condition")
  Compare To Constant8/1 -> Logical Operator11/1
  raptor_data_read6/1 -> Compare To Constant14/1, Compare To Constant15/1
  Compare To Constant9/1 -> Logical Operator11/2
  Warning8/1(Warning) -> raptor_data_write3/1
  Logical Operator13/1 -> Warning8/1(" condition")
  raptor_data_read8/1 -> Compare To Constant16/1, Compare To Constant17/1
  Compare To Constant17/1 -> Logical Operator13/2
  Compare To Constant16/1 -> Logical Operator13/1
  Compare To Constant23/1 -> Logical Operator14/2
  raptor_data_read10/1 -> Compare To Constant21/1, Compare To Constant20/1
  Compare To Constant22/1 -> Logical Operator14/1
  Logical Operator16/1 -> Warning9/1(" condition")
  Compare To Constant20/1 -> Logical Operator12/1
  Logical Operator14/1 -> Warning11/1(" condition")
  Logical Operator15/1 -> raptor_data_write4/1
  Warning10/1(Warning) -> Logical Operator15/2
  Compare To Constant21/1 -> Logical Operator12/2
  Warning9/1(Warning) -> Logical Operator15/1
  Logical Operator12/1 -> Warning10/1(" condition")
  Compare To Constant18/1 -> Logical Operator16/1
  Compare To Constant19/1 -> Logical Operator16/2
  raptor_data_read9/1 -> Compare To Constant19/1, Compare To Constant18/1
  raptor_data_read11/1 -> Compare To Constant23/1, Compare To Constant22/1
  Warning11/1(Warning) -> Logical Operator15/3
  Warning12/1(Warning) -> Logical Operator15/4
  raptor_data_read12/1 -> Compare To Constant24/1, Compare To Constant25/1
  Logical Operator17/1 -> Warning12/1(" condition")
  Compare To Constant24/1 -> Logical Operator17/1
  Compare To Constant25/1 -> Logical Operator17/2

== system EPT/Foreground_TimeBase_5ms/E//W /CAN_E//W/CAN_Fault ==
  BCU CAN Fault : Subsystem
  Compare To Constant4 : simulink/Logic and Bit Operations/Compare To Constant  relop===  const=1  OutDataTypeStr=boolean
  DCDC CAN Fault : Subsystem
  Detect Increase1 : simulink/Logic and Bit Operations/Detect Increase  vinit=0.0  OutDataTypeStr=boolean
  ECHS CAN Fault : Subsystem
  MCU CAN Fault : Subsystem
  OBC CAN Fault : Subsystem
  Reset Trigger : Subsystem
  raptor_adjustment1 : Raptor_lib/Data Storage/raptor_adjustment  paramName='Cal_Fault_Reset_Trigger'  nameSource=Parameter  initValue=0.00  dataType=boolean  storage=Calibration  calDispType=Number  calEnum={'False', 'True'}  calGain=1.0  calOffset=0.0  calMax=inf  calMin=-inf  calFormat='-1'  calUnit=''  calHelp=''  calAccess=1  calFunction=raptor_xcp_function(gcb)  calDispHeaders=off  calColHeaders={'Col1' 'Col2' 'Col3'}  calRowHeaders={'Row1' 'Row2' 'Row3'}
      settings: SourceProductName=Raptor
  raptor_adjustment2 : Raptor_lib/Data Storage/raptor_adjustment  paramName='Cal_Fault_Reset_Trigger_On'  nameSource=Parameter  initValue=0.00  dataType=boolean  storage=Calibration  calDispType=Number  calEnum={'False', 'True'}  calGain=1.0  calOffset=0.0  calMax=inf  calMin=-inf  calFormat='-1'  calUnit=''  calHelp=''  calAccess=1  calFunction=raptor_xcp_function(gcb)  calDispHeaders=off  calColHeaders={'Col1' 'Col2' 'Col3'}  calRowHeaders={'Row1' 'Row2' 'Row3'}
      settings: SourceProductName=Raptor
  raptor_data_def15 : Raptor_lib/Data Storage/raptor_data_def  dataName='Fault_Reset_Trigger'  initValue=0  dataType=boolean  storage=Volatile (RAM)  calVisible=on  calType=Measurement  calDispType=Number  calEnum={'False', 'True'}  calGain=1.0  calOffset=0  calMin=-inf  calMax=inf  calFormat='-1'  calUnit=''  calHelp=''  calAccess=1  calFunction=raptor_xcp_function(gcb)  calDispHeaders=off  calColHeaders={'Col1' 'Col2' 'Col3'}  calRowHeaders={'Row1' 'Row2' 'Row3'}
      settings: SourceProductName=Raptor
  raptor_data_read13 : Raptor_lib/Data Storage/raptor_data_read  dataName='Fault_Reset_Trigger'  dataShape=Scalar  idxSource=Input  idxRow=1  idxCol=1
      settings: SourceProductName=Raptor
  wires:
  Compare To Constant4/1 -> Detect Increase1/1
  raptor_adjustment1/1 -> Compare To Constant4/1
  Detect Increase1/1 -> Reset Trigger/1(Reset Trigger)
  raptor_adjustment2/1 -> Reset Trigger/Enable
  raptor_data_read13/1 -> OBC CAN Fault/1(Reset), DCDC CAN Fault/1(Reset), BCU CAN Fault/1(Reset), MCU CAN Fault/1(Reset), ECHS CAN Fault/1(Reset)

== system EPT/Foreground_TimeBase_5ms/E//W /E//W_Process/CAN_Fault ==
  Logical Operator4 : Logic  Operator=OR  Inputs=6  AllPortsSameDT=off  OutDataTypeStr=boolean
  raptor_data_read1 : Raptor_lib/Data Storage/raptor_data_read  dataName='CAN_Fault_IVT'  dataShape=Scalar  idxSource=Input  idxRow=1  idxCol=1
      settings: SourceProductName=Raptor
  raptor_data_read18 : Raptor_lib/Data Storage/raptor_data_read  dataName='CAN_Fault_MCU'  dataShape=Scalar  idxSource=Input  idxRow=1  idxCol=1
      settings: SourceProductName=Raptor
  raptor_data_read19 : Raptor_lib/Data Storage/raptor_data_read  dataName='CAN_Fault_CMU1'  dataShape=Scalar  idxSource=Input  idxRow=1  idxCol=1
      settings: SourceProductName=Raptor
  raptor_data_read2 : Raptor_lib/Data Storage/raptor_data_read  dataName='CAN_Fault_DCDC'  dataShape=Scalar  idxSource=Input  idxRow=1  idxCol=1
      settings: SourceProductName=Raptor
  raptor_data_read20 : Raptor_lib/Data Storage/raptor_data_read  dataName='CAN_Fault_CMU2'  dataShape=Scalar  idxSource=Input  idxRow=1  idxCol=1
      settings: SourceProductName=Raptor
  raptor_data_read3 : Raptor_lib/Data Storage/raptor_data_read  dataName='CAN_Fault_OBC'  dataShape=Scalar  idxSource=Input  idxRow=1  idxCol=1
      settings: SourceProductName=Raptor
  raptor_override1 : Raptor_lib/Data Storage/raptor_override  paramName='Cal_Bypass_CAN_Fault_MCU'  nameSource=Parameter  measurement=None  calDispType=Number  calEnum={'False', 'True'}  calGain=1.0  calOffset=0.0  calMax=inf  calMin=-inf  calFormat='-1'  calUnit=''  calHelp=''  calAccess=1  calFunction=[raptor_xcp_function(gcb) '|' raptor_get_param_eval(gcb, 'paramName') '_Override']
      settings: SourceProductName=Raptor
  raptor_override2 : Raptor_lib/Data Storage/raptor_override  paramName='Cal_Bypass_CAN_Fault_CMU1'  nameSource=Parameter  measurement=None  calDispType=Number  calEnum={'False', 'True'}  calGain=1.0  calOffset=0.0  calMax=inf  calMin=-inf  calFormat='-1'  calUnit=''  calHelp=''  calAccess=1  calFunction=[raptor_xcp_function(gcb) '|' raptor_get_param_eval(gcb, 'paramName') '_Override']
      settings: SourceProductName=Raptor
  raptor_override3 : Raptor_lib/Data Storage/raptor_override  paramName='Cal_Bypass_CAN_Fault_CMU2'  nameSource=Parameter  measurement=None  calDispType=Number  calEnum={'False', 'True'}  calGain=1.0  calOffset=0.0  calMax=inf  calMin=-inf  calFormat='-1'  calUnit=''  calHelp=''  calAccess=1  calFunction=[raptor_xcp_function(gcb) '|' raptor_get_param_eval(gcb, 'paramName') '_Override']
      settings: SourceProductName=Raptor
  raptor_override4 : Raptor_lib/Data Storage/raptor_override  paramName='Cal_Bypass_CAN_Fault_IVT'  nameSource=Parameter  measurement=None  calDispType=Number  calEnum={'False', 'True'}  calGain=1.0  calOffset=0.0  calMax=inf  calMin=-inf  calFormat='-1'  calUnit=''  calHelp=''  calAccess=1  calFunction=[raptor_xcp_function(gcb) '|' raptor_get_param_eval(gcb, 'paramName') '_Override']
      settings: SourceProductName=Raptor
  raptor_override5 : Raptor_lib/Data Storage/raptor_override  paramName='Cal_Bypass_CAN_Fault_DCDC'  nameSource=Parameter  measurement=None  calDispType=Number  calEnum={'False', 'True'}  calGain=1.0  calOffset=0.0  calMax=inf  calMin=-inf  calFormat='-1'  calUnit=''  calHelp=''  calAccess=1  calFunction=[raptor_xcp_function(gcb) '|' raptor_get_param_eval(gcb, 'paramName') '_Override']
      settings: SourceProductName=Raptor
  raptor_override6 : Raptor_lib/Data Storage/raptor_override  paramName='Cal_Bypass_CAN_Fault_OBC'  nameSource=Parameter  measurement=None  calDispType=Number  calEnum={'False', 'True'}  calGain=1.0  calOffset=0.0  calMax=inf  calMin=-inf  calFormat='-1'  calUnit=''  calHelp=''  calAccess=1  calFunction=[raptor_xcp_function(gcb) '|' raptor_get_param_eval(gcb, 'paramName') '_Override']
      settings: SourceProductName=Raptor
  Fault : Outport  VectorParamsAs1DForOutWhenUnconnected=off
  wires:
  raptor_data_read19/1 -> raptor_override2/1
  raptor_data_read20/1 -> raptor_override3/1
  raptor_data_read18/1 -> raptor_override1/1
  Logical Operator4/1 -> Fault/1
  raptor_data_read1/1 -> raptor_override4/1
  raptor_override1/1 -> Logical Operator4/1
  raptor_override2/1 -> Logical Operator4/2
  raptor_override3/1 -> Logical Operator4/3
  raptor_override4/1 -> Logical Operator4/4
  raptor_data_read2/1 -> raptor_override5/1
  raptor_data_read3/1 -> raptor_override6/1
  raptor_override5/1 -> Logical Operator4/5
  raptor_override6/1 -> Logical Operator4/6

== system EPT/Foreground_TimeBase_5ms/E//W /E//W_Process/ECHS_Fault ==
  Logical Operator : Logic  Operator=OR  AllPortsSameDT=off  OutDataTypeStr=boolean
  raptor_data_read1 : Raptor_lib/Data Storage/raptor_data_read  dataName='Flag_ECHS_Disconnected'  dataShape=Scalar  idxSource=Input  idxRow=1  idxCol=1
      settings: SourceProductName=Raptor
  raptor_data_read3 : Raptor_lib/Data Storage/raptor_data_read  dataName='ECHS_EW'  dataShape=Scalar  idxSource=Input  idxRow=1  idxCol=1
      settings: SourceProductName=Raptor
  raptor_override : Raptor_lib/Data Storage/raptor_override  paramName='Cal_Bypass_ECHS_Disconnected'  nameSource=Parameter  measurement=None  calDispType=Number  calEnum={'False', 'True'}  calGain=1.0  calOffset=0.0  calMax=inf  calMin=-inf  calFormat='-1'  calUnit=''  calHelp=''  calAccess=1  calFunction=[raptor_xcp_function(gcb) '|' raptor_get_param_eval(gcb, 'paramName') '_Override']
      settings: SourceProductName=Raptor
  raptor_override1 : Raptor_lib/Data Storage/raptor_override  paramName='Cal_Bypass_ECHS_EW'  nameSource=Parameter  measurement=None  calDispType=Number  calEnum={'False', 'True'}  calGain=1.0  calOffset=0.0  calMax=inf  calMin=-inf  calFormat='-1'  calUnit=''  calHelp=''  calAccess=1  calFunction=[raptor_xcp_function(gcb) '|' raptor_get_param_eval(gcb, 'paramName') '_Override']
      settings: SourceProductName=Raptor
  Fault : Outport  VectorParamsAs1DForOutWhenUnconnected=off
  wires:
  Logical Operator/1 -> Fault/1
  raptor_data_read3/1 -> raptor_override1/1
  raptor_data_read1/1 -> raptor_override/1
  raptor_override/1 -> Logical Operator/2
  raptor_override1/1 -> Logical Operator/1

== system EPT/Foreground_TimeBase_5ms/E//W /E//W_Process/OBU_Fault ==
  Bitwise Operator{,1..3} (4 alike) : simulink/Logic and Bit Operations/Bitwise Operator  logicop=AND  UseBitMask=off  NumInputPorts=2  BitMask=bin2dec('11011001')  BitMaskRealWorld=Stored Integer
  raptor_adjustment1 : Raptor_lib/Data Storage/raptor_adjustment  paramName='Cal_PB_OBU_G1_AND'  nameSource=Parameter  initValue=bin2dec('11111111')  dataType=uint8  storage=Calibration  calDispType=Number  calEnum={'False', 'True'}  calGain=1.0  calOffset=0.0  calMax=inf  calMin=-inf  calFormat='-1'  calUnit=''  calHelp=''  calAccess=1  calFunction=raptor_xcp_function(gcb)  calDispHeaders=off  calColHeaders={'Col1' 'Col2' 'Col3'}  calRowHeaders={'Row1' 'Row2' 'Row3'}
      settings: SourceProductName=Raptor
  raptor_adjustment2 : Raptor_lib/Data Storage/raptor_adjustment  paramName='Cal_PB_OBU_G2_AND'  nameSource=Parameter  initValue=bin2dec('11111111')  dataType=uint8  storage=Calibration  calDispType=Number  calEnum={'False', 'True'}  calGain=1.0  calOffset=0.0  calMax=inf  calMin=-inf  calFormat='-1'  calUnit=''  calHelp=''  calAccess=1  calFunction=raptor_xcp_function(gcb)  calDispHeaders=off  calColHeaders={'Col1' 'Col2' 'Col3'}  calRowHeaders={'Row1' 'Row2' 'Row3'}
      settings: SourceProductName=Raptor
  raptor_adjustment3 : Raptor_lib/Data Storage/raptor_adjustment  paramName='Cal_PB_OBU_G3_AND'  nameSource=Parameter  initValue=bin2dec('11111111')  dataType=uint8  storage=Calibration  calDispType=Number  calEnum={'False', 'True'}  calGain=1.0  calOffset=0.0  calMax=inf  calMin=-inf  calFormat='-1'  calUnit=''  calHelp=''  calAccess=1  calFunction=raptor_xcp_function(gcb)  calDispHeaders=off  calColHeaders={'Col1' 'Col2' 'Col3'}  calRowHeaders={'Row1' 'Row2' 'Row3'}
      settings: SourceProductName=Raptor
  raptor_adjustment4 : Raptor_lib/Data Storage/raptor_adjustment  paramName='Cal_PB_OBU_G4_AND'  nameSource=Parameter  initValue=bin2dec('01111111')  dataType=uint8  storage=Calibration  calDispType=Number  calEnum={'False', 'True'}  calGain=1.0  calOffset=0.0  calMax=inf  calMin=-inf  calFormat='-1'  calUnit=''  calHelp=''  calAccess=1  calFunction=raptor_xcp_function(gcb)  calDispHeaders=off  calColHeaders={'Col1' 'Col2' 'Col3'}  calRowHeaders={'Row1' 'Row2' 'Row3'}
      settings: SourceProductName=Raptor
  raptor_data_read1 : Raptor_lib/Data Storage/raptor_data_read  dataName='BP_OBU_Fault_G2'  dataShape=Scalar  idxSource=Input  idxRow=1  idxCol=1
      settings: SourceProductName=Raptor
  raptor_data_read17 : Raptor_lib/Data Storage/raptor_data_read  dataName='BP_OBU_Fault_G1'  dataShape=Scalar  idxSource=Input  idxRow=1  idxCol=1
      settings: SourceProductName=Raptor
  raptor_data_read2 : Raptor_lib/Data Storage/raptor_data_read  dataName='BP_OBU_Fault_G3'  dataShape=Scalar  idxSource=Input  idxRow=1  idxCol=1
      settings: SourceProductName=Raptor
  raptor_data_read4 : Raptor_lib/Data Storage/raptor_data_read  dataName='BP_OBU_Fault_G4'  dataShape=Scalar  idxSource=Input  idxRow=1  idxCol=1
      settings: SourceProductName=Raptor
  G1_Fault : Outport  VectorParamsAs1DForOutWhenUnconnected=off
  G2_Fault : Outport  Port=2  VectorParamsAs1DForOutWhenUnconnected=off
  G3_Fault : Outport  Port=3  VectorParamsAs1DForOutWhenUnconnected=off
  G4_Fault : Outport  Port=4  VectorParamsAs1DForOutWhenUnconnected=off
  wires:
  Bitwise Operator1/1 -> G2_Fault/1
  Bitwise Operator/1 -> G1_Fault/1
  Bitwise Operator3/1 -> G4_Fault/1
  Bitwise Operator2/1 -> G3_Fault/1
  raptor_data_read17/1 -> Bitwise Operator/2
  raptor_data_read1/1 -> Bitwise Operator1/2
  raptor_data_read2/1 -> Bitwise Operator2/2
  raptor_data_read4/1 -> Bitwise Operator3/2
  raptor_adjustment1/1 -> Bitwise Operator/1
  raptor_adjustment2/1 -> Bitwise Operator1/1
  raptor_adjustment3/1 -> Bitwise Operator2/1
  raptor_adjustment4/1 -> Bitwise Operator3/1

== system EPT/Foreground_TimeBase_5ms/OBP_Temp_Detection/CountTrigger/CycleTrigger ==
  In1 : Inport
  In2 : Inport  Port=2
  Add : Sum
  Add1 : Sum
  Add2 : Sum  Inputs=+-
  Constant1 : Constant
  Constant2 : Constant  Value=0
  Constant3 : Constant
  Data Type Conversion1 : DataTypeConversion
  Data Type Conversion2 : DataTypeConversion
  Display : Display
  Relational Operator1 : RelationalOperator  OutDataTypeStr=boolean  RndMeth=Simplest
  Scope : Scope
  Scope1 : Scope
  Scope2 : Scope
  Switch : Switch  Threshold=1
  Unit Delay : UnitDelay  SampleTime=-1  HasFrameUpgradeWarning=on
  Unit Delay1 : UnitDelay  SampleTime=-1  HasFrameUpgradeWarning=on
  Trigger : Outport  VectorParamsAs1DForOutWhenUnconnected=off
  wires:
  Add/1 -> Switch/1
  In1/1 -> Data Type Conversion2/1
  Unit Delay/1 -> Add/1
  Switch/1 -> Relational Operator1/1, Scope1/1, Unit Delay/1
  Add1/1 -> Scope/1, Unit Delay1/1, Display/1
  Unit Delay1/1 -> Add1/1
  Constant1/1 -> Add1/2
  Relational Operator1/1 -> Scope2/1, Trigger/1
  Data Type Conversion1/1 -> Relational Operator1/2
  Constant2/1 -> Switch/3
  Data Type Conversion2/1 -> Add/2, Switch/2
  Add2/1 -> Data Type Conversion1/1
  In2/1 -> Add2/1
  Constant3/1 -> Add2/2
